simulink model "kalman2"  (R2022b)
settings: Solver=FixedStepAuto  StartTime=0.0  StopTime=10.0  FixedStep=0.0001  RelTol=1e-3
values from neighbouring files (symbols this model uses):
  A = [0 1 0; a21 0 a23; a31 0 a33]    [ex6.m]    (also in kf.m)
  B = [0 0; 0 g; b31 0]    [ex6.m]    (also in kf.m)
  C = [1 0 0]    [ex6.m]    (also in kf.m)
  Kx = -acker(A, B(:,1), -sKx)    [ex6.m]
  xd = d-bd    (= 0.0192)    [ex6.m]    (also in kf.m)
settings Model: Creator=AgraWoodAdmin  LastModifiedBy=AgraWoodAdmin

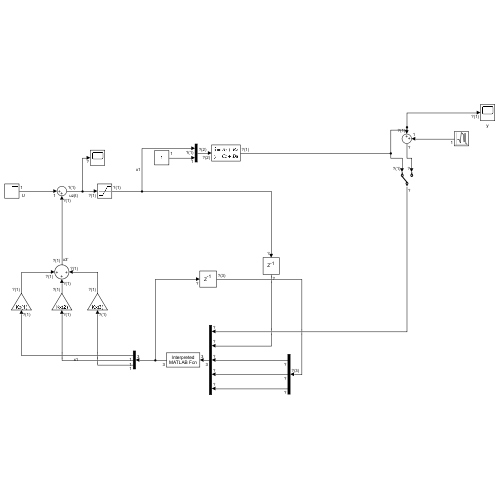
[thumbnail: Simulink's stored preview of the top-level diagram]
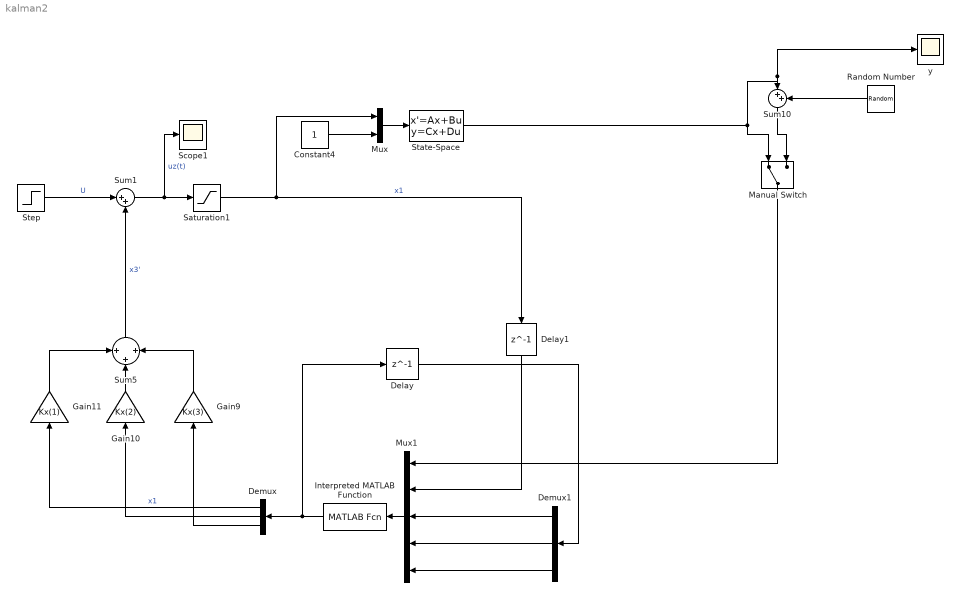
== system kalman2 ==
  Constant4 : Constant
  Delay : Delay  DelayLength=1  InitialCondition=[xd; 0; 0]
  Delay1 : Delay  DelayLength=1
  Demux : Demux  Outputs=3
  Demux1 : Demux  Outputs=3
  Gain10 : Gain  Gain=Kx(2)
  Gain11 : Gain  Gain=Kx(1)
  Gain9 : Gain  Gain=Kx(3)
  Interpreted MATLAB Function : MATLABFcn
  Manual Switch : ManualSwitch
  Mux : Mux  Inputs=2
  Mux1 : Mux  Inputs=5
  Random Number : RandomNumber  Variance=.0000001
  Saturation1 : Saturate  UpperLimit=1  LowerLimit=0
  Scope1 : Scope
  State-Space : StateSpace  A=A  B=B  C=C  D=[0 0]  InitialCondition=[xd; 0; 0]
  Step : Step  Time=0  SampleTime=0
  Sum1 : Sum  Inputs=|++
  Sum10 : Sum  Inputs=|++
  Sum5 : Sum  Inputs=+|+|+
  y : Scope
  wires:
  Demux/3 -> Gain9/1
  Gain9/1 -> Sum5/3
  Sum1/1 -> Saturation1/1, Scope1/1  "uz(t)"
  Demux/2 -> Gain10/1
  Saturation1/1 -> Mux/1, Delay1/1  "x1"
  Sum5/1 -> Sum1/2  "x3'"
  Gain10/1 -> Sum5/2
  Sum10/1 -> Manual Switch/2
  Step/1 -> Sum1/1  "U"
  Demux/1 -> Gain11/1  "x1"
  Gain11/1 -> Sum5/1
  Mux/1 -> State-Space/1
  Manual Switch/1 -> Mux1/1
  Delay1/1 -> Mux1/2
  State-Space/1 -> y/1, Sum10/1, Manual Switch/1
  Random Number/1 -> Sum10/2
  Constant4/1 -> Mux/2
  Delay/1 -> Demux1/1
  Mux1/1 -> Interpreted MATLAB Function/1
  Demux1/3 -> Mux1/5
  Demux1/2 -> Mux1/4
  Demux1/1 -> Mux1/3
  Interpreted MATLAB Function/1 -> Delay/1, Demux/1
